simulink model "Temporal2_2018a"  (R2018a)
settings: Solver=FixedStepDiscrete  StartTime=0.0  StopTime=20  FixedStep=0.1  RelTol=1e-3  EnableMultiTasking=on
settings Model: Creator=bzhan  LastModifiedBy=bzhan
settings SolverCC: AutoInsertRateTranBlk=on
settings DataIOCC: LimitDataPoints=on  ReturnWorkspaceOutputs=on
settings OptimizationCC: LifeSpan=inf
settings DebuggingCC: AllowSymbolicDim=off  SFUnexpectedBacktrackingDiag=warning  SFNoUnconditionalDefaultTransitionDiag=warning  SFExecutionAtInitializationDiag=none
settings CodeAppCC: StateflowObjectComments=on
settings GRTTargetCC: TargetLangStandard=C89/C90 (ANSI)
settings ConfigComp: CovMetricSettings=dw  CovHtmlReporting=on  CovSaveCumulativeToWorkspaceVar=on  CovSaveSingleToWorkspaceVar=on  CovShowResultsExplorer=off  CovExternalEMLEnable=off  CovSFcnEnable=off

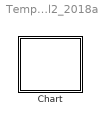
== system Temporal2_2018a ==
  Chart : Stateflow chart  TreatAsAtomicUnit=on

== stateflow chart Temporal2_2018a/Chart ==
  settings: updateMethod=DISCRETE  sampleTime=1
  state A
    en: f("en_A"); ra=random();
  state B
    en: f("en_B"); rb=random();
  (default) -> A
  A -> B : after(ra,sec)
  B -> A : after(rb,sec)
  data: s function_input; r function_output; ra local; rb local
  function f(s):
    | function f(s)
    |   fprintf(s+"\n");
  function r = random:
    | function r = random
    |   r = unidrnd(5);
    |   fprintf("Picked %.0f\n", r);
